simulink model "traj_player"  (R2022b)
settings: Solver=VariableStepAuto  StartTime=0.0  StopTime=8  RelTol=1e-3
values from neighbouring files (symbols this model uses):
  leg_model_obj = leg_model    [initialize_sim_parameters.m]    (also in pos_control_setup.m)
  N = 30    [pos_control_setup.m]    (also in traj_player_prepar.m = 150)
  nu = 3    [pos_control_setup.m]    (also in traj_player_prepar.m)
  nx = 10    [pos_control_setup.m]    (also in traj_player_prepar.m)
  nx_l = 10    [initialize_sim_parameters.m]    (also in pos_control_setup.m)
  Th = 1.5    [pos_control_setup.m]    (also in traj_player_prepar.m = 0.75)
  u_ref = zeros(3*N,1)    [traj_player_prepar.m]
  x_ref = zeros(10*(N+1),1)    [traj_player_prepar.m]
undefined symbols (not defined in the file or in its folder): Kd, Kp
libraries: slpidlib x4
settings Model: Creator=papaveneti  LastModifiedBy=papaveneti

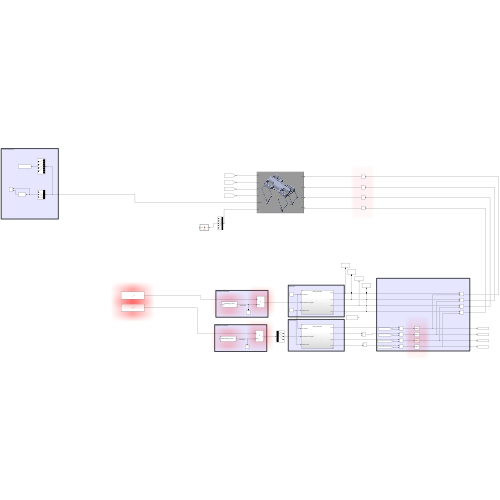
[thumbnail: Simulink's stored preview of the top-level diagram]
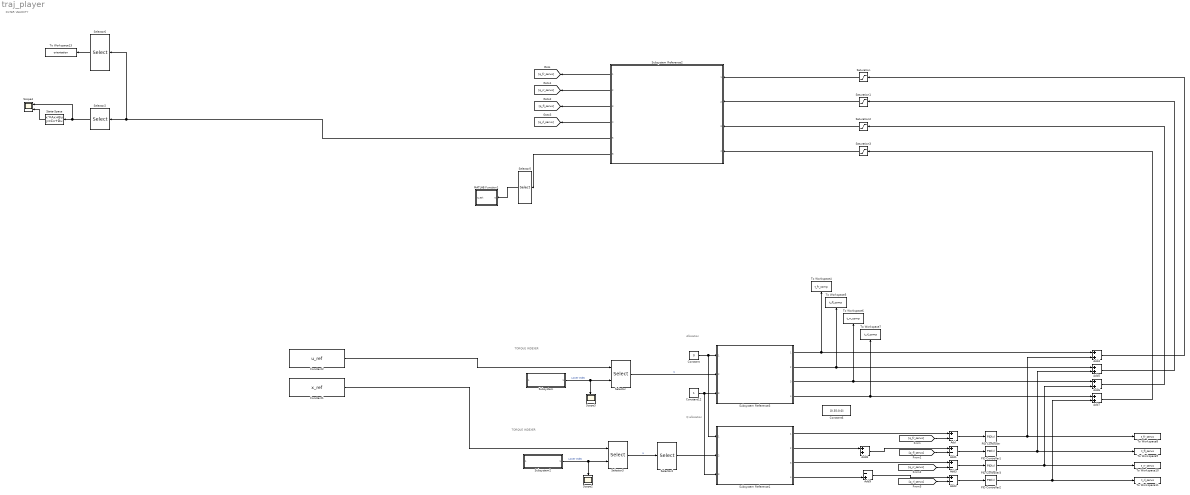
== system traj_player ==
  note: TORQUE INDEXER
  note: Q allocation
  note: Allocation
  note: TORQUE INDEXER
  note: FILTER VELOCITY
  Add{,1..3} (4 alike) : Sum  Inputs=+-
  Add{4..8} (5 alike) : Sum
  Add9 : Sum  Inputs=-+
  Constant : Constant  Value=0
  Constant1 : Constant  Value=x_ref
  Constant12 : Constant
  Constant2 : Constant  Value=u_ref
  Constant6 : Constant  Value=[0.35;0;0]
  MATLAB Function1 : MATLAB Function  TreatAsAtomicUnit=on
  PID Controller{,1..3} (4 alike) : slpidlib/PID Controller  Controller=PID  Form=Parallel  TimeDomain=Discrete-time  UseExternalTs=off  SampleTime=-1  IntegratorMethod=Forward Euler  FilterMethod=Forward Euler  ControllerParametersSource=internal  P=Kp  I=0  UseKiTs=off  D=Kd  N=100  UseFilter=on  TunerSelectOption=Transfer Function Based (PID Tuner App)  InitialConditionSource=internal  InitialConditionForIntegrator=0  InitialConditionForFilter=0  DifferentiatorICPrevScaledInput=0  ExternalReset=none  TrackingMode=off  Kt=1  LimitOutput=off  SatLimitsSource=internal  UpperSaturationLimit=inf  LowerSaturationLimit=-inf  LinearizeAsGain=on  AntiWindupMode=none  Kb=1  LimitIntegrator=off  UpperIntegratorSaturationLimit=inf  LowerIntegratorSaturationLimit=-inf  POutMin=[]  POutMax=[]  IOutMin=[]  IOutMax=[]  DOutMin=[]  DOutMax=[]  NOutMin=[]  NOutMax=[]  SumOutMin=[]  SumOutMax=[]  SaturationOutMin=[]  SaturationOutMax=[]  PParamMin=[]  PParamMax=[]  IParamMin=[]  IParamMax=[]  DParamMin=[]  DParamMax=[]  NParamMin=[]  NParamMax=[]  KbParamMin=[]  KbParamMax=[]  KtParamMin=[]  KtParamMax=[]  KbOutMin=[]  KbOutMax=[]  KtOutMin=[]  KtOutMax=[]  IntegratorOutMin=[]  IntegratorOutMax=[]  FilterOutMin=[]  FilterOutMax=[]  SumI1OutMin=[]  SumI1OutMax=[]  SumI2OutMin=[]  SumI2OutMax=[]  SumI3OutMin=[]  SumI3OutMax=[]  SumI4OutMin=[]  SumI4OutMax=[]  SumDOutMin=[]  SumDOutMax=[]  DifferentiatorOutMin=[]  DifferentiatorOutMax=[]  FilterDiffOutCoefMin=[]  FilterDiffOutCoefMax=[]  ReciprocalOutMin=[]  ReciprocalOutMax=[]  SumDenOutMin=[]  SumDenOutMax=[]  SumNumOutMin=[]  SumNumOutMax=[]  DivideOutMin=[]  DivideOutMax=[]  UdiffTsProdOutMin=[]  UdiffTsProdOutMax=[]  NTsProdOutMin=[]  NTsProdOutMax=[]  UintegralTsProdOutMin=[]  UintegralTsProdOutMax=[]  UngainTsProdOutMin=[]  UngainTsProdOutMax=[]  ClampingZeroOutDataTypeStr=Inherit: Inherit via back propagation  ClampingZeroOutMin=[]  ClampingZeroOutMax=[]  FilterDenConstantOutDataTypeStr=Inherit: Inherit via back propagation  FilterDenConstantOutMin=[]  FilterDenConstantOutMax=[]  PCopyOutDataTypeStr=Inherit: Inherit via back propagation  PCopyOutMin=[]  PCopyOutMax=[]  NCopyOutDataTypeStr=Inherit: Inherit via back propagation  NCopyOutMin=[]  NCopyOutMax=[]  IntegratorContinuousStateAttributes=''  IntegratorStateMustResolveToSignalObject=off  IntegratorRTWStateStorageClass=Auto  FilterContinuousStateAttributes=''  FilterStateMustResolveToSignalObject=off  FilterRTWStateStorageClass=Auto  ParallelPVariant=InternalParameters  IdealPVariant=Disabled  IVariant=InternalParameters  DVariant=InternalParameters  IntegratorVariant=Discrete  SatVariant=Disabled  AWVariant=Passthrough  PCopyVariant=Disabled  TRVariant=Disabled  FdbkBlocksVariant=Forward  IdealPFdbkVariant=Disabled  SatFdbkVariant=Disabled  DerivativeFilterVariant=ForwardEulerFilter  NVariant=InternalParameters  NCopyVariant=Disabled  FilterICVariant=InternalICsFilter  IntegratorICVariant=InternalICs  ExternalResetVariant=Disabled  TRSumVariant=Passthrough  SumFdbkVariant=Disabled  SumVariant=Sum_PID  TsampFilterVariant=InternalTs  TsampNgainVariant=Passthrough  TsampIntegralVariant=Passthrough  ExternalSaturationOutDataTypeStr=Inherit: Same as second input
  Saturation{,1..3} (4 alike) : Saturate  UpperLimit=leg_model_obj.input_constraints(:,2)  LowerLimit=leg_model_obj.input_constraints(:,1)
  Scope2 : Scope
  Scope3 : Scope
  Scope4 : Scope  NumInputPorts=2
  Selector : Selector  InputPortWidth=N*nu  IndexOptions=Starting index (port)  Indices=[1 3]  OutputSizes=nu_l
  Selector2 : Selector  InputPortWidth=7  IndexOptions=Index vector (dialog)  Indices=[5:7]  OutputSizes=1
  Selector3 : Selector  InputPortWidth=(N+1)*nx  IndexOptions=Starting index (port)  Indices=[1 3]  OutputSizes=nx_l
  Selector4 : Selector  InputPortWidth=10  IndexOptions=Index vector (dialog)  Indices=[1,2,4]  OutputSizes=1
  Selector5 : Selector  InputPortWidth=10  IndexOptions=Starting index (dialog)  Indices=1  OutputSizes=5
  Selector6 : Selector  InputPortWidth=7  IndexOptions=Index vector (dialog)  Indices=[1,2,3,4]  OutputSizes=1
  State-Space : StateSpace  A=diag([-5,-5,-5])  B=2*eye(3)  C=2.5*eye(3)  D=zeros(3,3)  InitialCondition=0
  Subsystem : Subsystem  ReferencedSubsystem=overflowing_counter  Td=Th/N  Overflow_point=N*nu  Increment=nu
  Subsystem Reference1 : Subsystem  ReferencedSubsystem=torque_allocation
  Subsystem Reference2 : Subsystem  ReferencedSubsystem=olympus
  Subsystem Reference3 : Subsystem  ReferencedSubsystem=torque_allocation
  Subsystem2 : Subsystem  ReferencedSubsystem=overflowing_counter  Td=Th/N  Overflow_point=nx*N  Increment=nx_l
  To Workspace10 : ToWorkspace  VariableName=t_rr_servo  SaveFormat=Timeseries  SampleTime=-1
  To Workspace11 : ToWorkspace  VariableName=t_rl_servo  SaveFormat=Timeseries  SampleTime=-1
  To Workspace13 : ToWorkspace  VariableName=orientation  SaveFormat=Timeseries  SampleTime=-1
  To Workspace4 : ToWorkspace  VariableName=t_fr_comp  SaveFormat=Timeseries  SampleTime=-1
  To Workspace5 : ToWorkspace  VariableName=t_fl_comp  SaveFormat=Timeseries  SampleTime=-1
  To Workspace6 : ToWorkspace  VariableName=t_rr_comp  SaveFormat=Timeseries  SampleTime=-1
  To Workspace7 : ToWorkspace  VariableName=t_rl_comp  SaveFormat=Timeseries  SampleTime=-1
  To Workspace8 : ToWorkspace  VariableName=t_fr_servo  SaveFormat=Timeseries  SampleTime=-1
  To Workspace9 : ToWorkspace  VariableName=t_fl_servo  SaveFormat=Timeseries  SampleTime=-1
  wires:
  Subsystem/1 -> Selector/2, Scope3/1  "Lower Index"
  Subsystem Reference3/4 -> Add7/1, To Workspace7/1
  Subsystem Reference2/2 -> [q_rr_servo]
  Saturation2/1 -> Subsystem Reference2/3
  Subsystem Reference2/1 -> [q_fr_servo]
  Saturation3/1 -> Subsystem Reference2/4
  PID Controller1/1 -> To Workspace9/1, Add5/2
  Subsystem Reference1/1 -> Add/1
  Add4/1 -> Saturation/1
  [q_rl_servo] -> Add2/2
  Subsystem Reference3/1 -> Add4/1, To Workspace4/1
  Add9/1 -> Add2/1
  Constant2/1 -> Selector/1
  Selector3/1 -> Selector4/1  "U"
  Selector/1 -> Subsystem Reference3/2  "U"
  PID Controller3/1 -> To Workspace10/1, Add6/2
  Subsystem2/1 -> Scope2/1, Selector3/2  "Lower Index"
  Saturation1/1 -> Subsystem Reference2/2
  Subsystem Reference2/4 -> [q_rl_servo]
  PID Controller2/1 -> Add7/2, To Workspace11/1
  Add/1 -> PID Controller/1
  Constant12/1 -> Subsystem Reference1/3, Subsystem Reference3/3
  Add7/1 -> Saturation3/1
  Constant1/1 -> Selector3/1
  Selector4/1 -> Subsystem Reference1/2
  Add3/1 -> PID Controller3/1
  Saturation/1 -> Subsystem Reference2/1
  Selector5/1 -> MATLAB Function1/1(q)
  Subsystem Reference2/3 -> [q_fl_servo]
  [q_fl_servo] -> Add1/2
  Subsystem Reference3/2 -> Add5/1, To Workspace5/1
  Constant/1 -> Subsystem Reference1/1, Subsystem Reference3/1
  Add1/1 -> PID Controller1/1
  PID Controller/1 -> To Workspace8/1, Add4/2
  [q_fr_servo] -> Add/2
  Subsystem Reference1/2 -> Add8/1
  Subsystem Reference2/6 -> Selector5/1
  Add2/1 -> PID Controller2/1
  Subsystem Reference2/5 -> Selector6/1, Selector2/1
  [q_rr_servo] -> Add3/2
  Add8/1 -> Add1/1
  Subsystem Reference1/3 -> Add3/1
  Subsystem Reference1/4 -> Add9/2
  Subsystem Reference3/3 -> Add6/1, To Workspace6/1
  Add5/1 -> Saturation1/1
  Add6/1 -> Saturation2/1
  State-Space/1 -> Scope4/2
  Selector2/1 -> State-Space/1, Scope4/1
  Selector6/1 -> To Workspace13/1

== matlab function traj_player/MATLAB Function1 ==
  data: q input size=5; q_est output
function q_est = DK(q)
%% defines
qMH_offset = -pi/2;
q11_offset = 2.3095;
q21_offset = 1.3265;
q12_offset = 0.83482;
q22_offset = -1.3233;

j11_Dx = 0.046; %Horizontal distance of joint11 from MH frame
l11    = 0.18;
l21    = 0.29977;

j12_Dx = 0.136; %Horizontal distance of joint12 from MH frame
l12    = 0.18;
l22    = 0.29929;

j_Dy = -1.1338e-05; %Vertical Distance of joint11 and joint12 from MH frame
pj11 = [0.046, -1.1338e-05]; % `pj11` is the center of joint11
pj12 = [0.136, -1.1338e-05]; % `pj12` is the center of joint12 
%% Intersection point
p1c = zeros(1,2);
p2c = zeros(1,2);


q11 = -q(2) + q11_offset;
q12 = -q(4) + q12_offset;

%centers
p1c(1) = j11_Dx + l11*cos(q11);
p1c(2) = j_Dy   + l11*sin(q11);

p2c(1) = j12_Dx + l12*cos(q12);
p2c(2) = j_Dy   + l12*sin(q12);

% normal and center vector
vc = p2c-p1c;
d  = norm(vc); %distance of circle centers `p1c` and `p2c`
vc = vc/d;
vn = [-vc(2),vc(1)];

%%triangle solution
a = ( (d*d) + (l21*l21) - (l22*l22) )/( 2*d );
h = sqrt( (l21*l21) - (a*a));

p_EE_22d = p1c + (a*vc) + (h*vn);


%% joint angles
link11_v = p1c-pj11;
link12_v = p2c-pj12;

link21_v = p_EE_22d-p1c;
link22_v = p_EE_22d-p2c;

theta1 = acos(dot(link11_v, link21_v) / (norm(link11_v) * norm(link21_v)));
theta2 = -acos(dot(link12_v, link22_v) / (norm(link12_v) * norm(link22_v)));

% Check direction
link11_vn = link11_v / norm(link11_v);
side1_extended_x = link11_vn(1) * (l11 + l21);

link12_vn = link12_v / norm(link12_v);
side2_extended_x = link12_vn(1) * (l12 + l22);

%This can happen -> but i will not pass it in MPC
% if p_EE_22d(1) < side1_extended_x
%     % joint12 is outwards
%     theta1 = -theta1;
% elseif p_EE_22d(1) > side2_extended_x
%     % joint22 is outwards
%     theta2 = -theta2;
% end


q_est    = zeros(5,1);
q_est(1) = q(1);
q_est(2) = q(2);
q_est(3) = theta1 - q21_offset;
q_est(4) = q(4);
q_est(5) = theta2 - q22_offset;

end
